simulink model "model_5"  (R2017b)
settings: Solver=ode3  StartTime=0.0  StopTime=4  FixedStep=2e-6  MaxStep=2e-05  RelTol=1e-3
undefined symbols (not defined in the file or in its folder): c1, c2_dot, c3_dot, c4_dot, J_10_dot, J_1_dot, J_2_dot, J_37_dot, J_810_dot, M_51new, M_52new, Mdnew, Mf10_mass5, Mf1_mass5, Mf2_mass5, Mf37_mass5, Mf810_mass5
libraries: fl_lib x29, nesl_utility x11, simulink x5
settings Model: Creator=Elena  LastModifiedBy=Elena
settings SolverCC: ZeroCrossAlgorithm=Adaptive
settings DebuggingCC: IgnoredZcDiagnostic=none
settings CodeAppCC: StateflowObjectComments=on

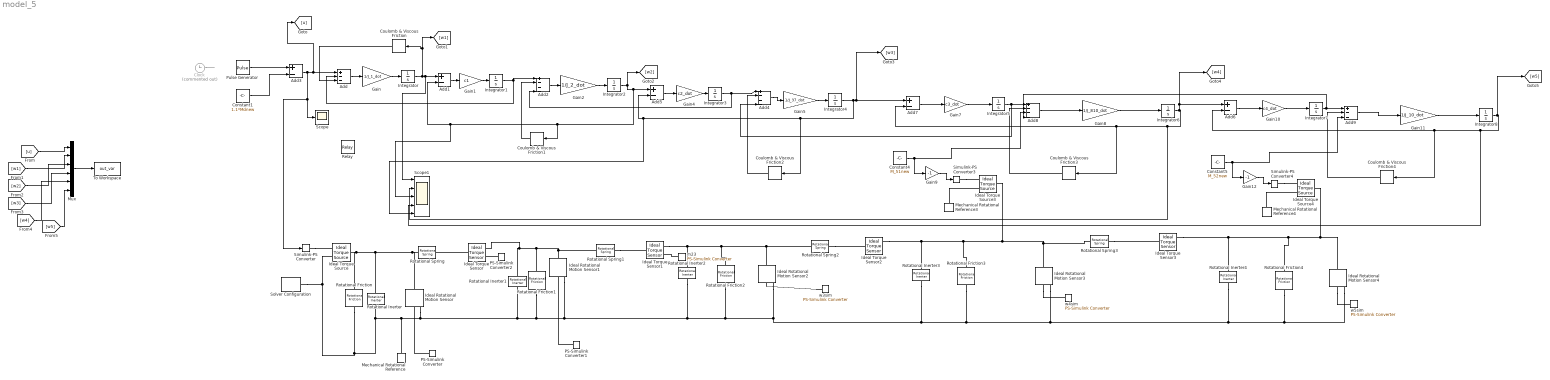
== system model_5 ==
  Add : Sum  Inputs=+--
  Add{1,3,5..7} (5 alike) : Sum  Inputs=+-
  Add2 : Sum  Inputs=+---
  Add4 : Sum  Inputs=+---
  Add8 : Sum  Inputs=+---
  Add9 : Sum  Inputs=+--
  Clock : Clock  Commented=on
  Constant1 : Constant  Value=1.1*Mdnew
  Constant4 : Constant  Value=M_51new
  Constant5 : Constant  Value=M_52new
  Coulomb & Viscous Friction : simulink/Discontinuities/Coulomb & Viscous Friction  offset=[Mf1_mass5]  gain=0
      settings: SourceProductName=Simulink
  Coulomb & Viscous Friction1 : simulink/Discontinuities/Coulomb & Viscous Friction  offset=[Mf2_mass5]  gain=0
      settings: SourceProductName=Simulink
  Coulomb & Viscous Friction2 : simulink/Discontinuities/Coulomb & Viscous Friction  offset=[Mf37_mass5]  gain=0
      settings: SourceProductName=Simulink
  Coulomb & Viscous Friction3 : simulink/Discontinuities/Coulomb & Viscous Friction  offset=[Mf810_mass5]  gain=0
      settings: SourceProductName=Simulink
  Coulomb & Viscous Friction4 : simulink/Discontinuities/Coulomb & Viscous Friction  offset=[Mf10_mass5]  gain=0
      settings: SourceProductName=Simulink
  Gain : Gain  Gain=1/J_1_dot
  Gain1 : Gain  Gain=c1
  Gain10 : Gain  Gain=c4_dot
  Gain11 : Gain  Gain=1/J_10_dot
  Gain12 : Gain  Gain=-1
  Gain2 : Gain  Gain=1/J_2_dot
  Gain4 : Gain  Gain=c2_dot
  Gain5 : Gain  Gain=1/J_37_dot
  Gain7 : Gain  Gain=c3_dot
  Gain8 : Gain  Gain=1/J_810_dot
  Gain9 : Gain  Gain=-1
  Ideal Rotational Motion Sensor{,1..4} (5 alike) : fl_lib/Mechanical/Mechanical Sensors/Ideal Rotational Motion Sensor  offset=0 rad
      settings: SourceProductBaseCode=PW,SS,VE
  Ideal Torque Sensor{,1..3} (4 alike) : fl_lib/Mechanical/Mechanical Sensors/Ideal Torque Sensor
      settings: SourceProductBaseCode=PW,SS,VE
  Ideal Torque Source : fl_lib/Mechanical/Mechanical Sources/Ideal Torque Source
      settings: SourceProductBaseCode=PW,SS,VE
  Ideal Torque Source3 : fl_lib/Mechanical/Mechanical Sources/Ideal Torque Source
      settings: SourceProductBaseCode=PW,SS,VE
  Ideal Torque Source4 : fl_lib/Mechanical/Mechanical Sources/Ideal Torque Source
      settings: SourceProductBaseCode=PW,SS,VE
  Integrator{,1..8} (9 alike) : Integrator
  Mechanical Rotational Reference : fl_lib/Mechanical/Rotational Elements/Mechanical Rotational Reference
      settings: SourceProductBaseCode=PW,SS,VE
  Mechanical Rotational Reference3 : fl_lib/Mechanical/Rotational Elements/Mechanical Rotational Reference
      settings: SourceProductBaseCode=PW,SS,VE
  Mechanical Rotational Reference4 : fl_lib/Mechanical/Rotational Elements/Mechanical Rotational Reference
      settings: SourceProductBaseCode=PW,SS,VE
  Mux : Mux  Inputs=6
  PS-Simulink Converter : nesl_utility/PS-Simulink Converter  PhysicalDomain=network_engine_domain  SubClassName=ps_output  LeftPortType=input  RightPortType=output  PseudoPeriodic=off  Frequencies=[]  Unit=rad/s  AffineConversion=off
      settings: SourceProductBaseCode=SS,PW,VE
  PS-Simulink Converter1 : nesl_utility/PS-Simulink Converter  PhysicalDomain=network_engine_domain  SubClassName=ps_output  LeftPortType=input  RightPortType=output  PseudoPeriodic=off  Frequencies=[]  Unit=rad/s  AffineConversion=off
      settings: SourceProductBaseCode=SS,PW,VE
  PS-Simulink Converter2 : nesl_utility/PS-Simulink Converter  PhysicalDomain=network_engine_domain  SubClassName=ps_output  LeftPortType=input  RightPortType=output  PseudoPeriodic=off  Frequencies=[]  Unit=N*m  AffineConversion=off
      settings: SourceProductBaseCode=SS,PW,VE
  Pulse Generator : DiscretePulseGenerator  PulseType=Time based  Amplitude=2.2*Mdnew  Period=1  PulseWidth=50
  Relay : Relay
  Rotational Friction : fl_lib/Mechanical/Rotational Elements/Rotational Friction  brkwy_trq=Mf1_mass5 N*m  brkwy_vel=1e-06 rad/s  Col_trq=Mf1_mass5 N*m  visc_coef=0 N*m/(rad/s)  w_specify=off  w_priority=None  w=0 rad/s  w_nominal_specify=off  w_nominal_unit=rad/s  w_nominal_value=1  t_specify=off  t_priority=None  t=0 N*m  t_nominal_specify=off  t_nominal_unit=N*m  t_nominal_value=1
      settings: SourceProductBaseCode=PW,SS,VE
  Rotational Friction1 : fl_lib/Mechanical/Rotational Elements/Rotational Friction  brkwy_trq=Mf2_mass5 N*m  brkwy_vel=1e-06 rad/s  Col_trq=Mf2_mass5 N*m  visc_coef=0 N*m/(rad/s)  w_specify=off  w_priority=None  w=0 rad/s  w_nominal_specify=off  w_nominal_unit=rad/s  w_nominal_value=1  t_specify=off  t_priority=None  t=0 N*m  t_nominal_specify=off  t_nominal_unit=N*m  t_nominal_value=1
      settings: SourceProductBaseCode=PW,SS,VE
  Rotational Friction2 : fl_lib/Mechanical/Rotational Elements/Rotational Friction  brkwy_trq=Mf37_mass5 N*m  brkwy_vel=1e-06 rad/s  Col_trq=Mf37_mass5 N*m  visc_coef=0 N*m/(rad/s)  w_specify=off  w_priority=None  w=0 rad/s  w_nominal_specify=off  w_nominal_unit=rad/s  w_nominal_value=1  t_specify=off  t_priority=None  t=0 N*m  t_nominal_specify=off  t_nominal_unit=N*m  t_nominal_value=1
      settings: SourceProductBaseCode=PW,SS,VE
  Rotational Friction3 : fl_lib/Mechanical/Rotational Elements/Rotational Friction  brkwy_trq=Mf810_mass5 N*m  brkwy_vel=1e-06 rad/s  Col_trq=Mf810_mass5 N*m  visc_coef=0 N*m/(rad/s)  w_specify=off  w_priority=None  w=0 rad/s  w_nominal_specify=off  w_nominal_unit=rad/s  w_nominal_value=1  t_specify=off  t_priority=None  t=0 N*m  t_nominal_specify=off  t_nominal_unit=N*m  t_nominal_value=1
      settings: SourceProductBaseCode=PW,SS,VE
  Rotational Friction4 : fl_lib/Mechanical/Rotational Elements/Rotational Friction  brkwy_trq=Mf10_mass5 N*m  brkwy_vel=1e-06 rad/s  Col_trq=Mf10_mass5 N*m  visc_coef=0 N*m/(rad/s)  w_specify=off  w_priority=None  w=0 rad/s  w_nominal_specify=off  w_nominal_unit=rad/s  w_nominal_value=1  t_specify=off  t_priority=None  t=0 N*m  t_nominal_specify=off  t_nominal_unit=N*m  t_nominal_value=1
      settings: SourceProductBaseCode=PW,SS,VE
  Rotational Inerter : fl_lib/Mechanical/Rotational Elements/Rotational Inerter  B=J_1_dot kg*m^2  w_specify=off  w_priority=High  w=0 rad/s  w_nominal_specify=off  w_nominal_unit=rad/s  w_nominal_value=1  t_specify=off  t_priority=None  t=0 N*m  t_nominal_specify=off  t_nominal_unit=N*m  t_nominal_value=1
      settings: SourceProductBaseCode=PW,SS,VE
  Rotational Inerter1 : fl_lib/Mechanical/Rotational Elements/Rotational Inerter  B=J_2_dot kg*m^2  w_specify=off  w_priority=High  w=0 rad/s  w_nominal_specify=off  w_nominal_unit=rad/s  w_nominal_value=1  t_specify=off  t_priority=None  t=0 N*m  t_nominal_specify=off  t_nominal_unit=N*m  t_nominal_value=1
      settings: SourceProductBaseCode=PW,SS,VE
  Rotational Inerter2 : fl_lib/Mechanical/Rotational Elements/Rotational Inerter  B=J_37_dot kg*m^2  w_specify=off  w_priority=High  w=0 rad/s  w_nominal_specify=off  w_nominal_unit=rad/s  w_nominal_value=1  t_specify=off  t_priority=None  t=0 N*m  t_nominal_specify=off  t_nominal_unit=N*m  t_nominal_value=1
      settings: SourceProductBaseCode=PW,SS,VE
  Rotational Inerter3 : fl_lib/Mechanical/Rotational Elements/Rotational Inerter  B=J_810_dot kg*m^2  w_specify=off  w_priority=High  w=0 rad/s  w_nominal_specify=off  w_nominal_unit=rad/s  w_nominal_value=1  t_specify=off  t_priority=None  t=0 N*m  t_nominal_specify=off  t_nominal_unit=N*m  t_nominal_value=1
      settings: SourceProductBaseCode=PW,SS,VE
  Rotational Inerter4 : fl_lib/Mechanical/Rotational Elements/Rotational Inerter  B=J_10_dot kg*m^2  w_specify=off  w_priority=High  w=0 rad/s  w_nominal_specify=off  w_nominal_unit=rad/s  w_nominal_value=1  t_specify=off  t_priority=None  t=0 N*m  t_nominal_specify=off  t_nominal_unit=N*m  t_nominal_value=1
      settings: SourceProductBaseCode=PW,SS,VE
  Rotational Spring : fl_lib/Mechanical/Rotational Elements/Rotational Spring  spr_rate=c1 N*m/rad  w_specify=off  w_priority=None  w=0 rad/s  w_nominal_specify=off  w_nominal_unit=rad/s  w_nominal_value=1  t_specify=off  t_priority=None  t=0 N*m  t_nominal_specify=off  t_nominal_unit=N*m  t_nominal_value=1  phi_specify=off  phi_priority=High  phi=0 rad  phi_nominal_specify=off  phi_nominal_unit=rad  phi_nominal_value=1
      settings: SourceProductBaseCode=PW,SS,VE
  Rotational Spring1 : fl_lib/Mechanical/Rotational Elements/Rotational Spring  spr_rate=c2_dot N*m/rad  w_specify=off  w_priority=None  w=0 rad/s  w_nominal_specify=off  w_nominal_unit=rad/s  w_nominal_value=1  t_specify=off  t_priority=None  t=0 N*m  t_nominal_specify=off  t_nominal_unit=N*m  t_nominal_value=1  phi_specify=off  phi_priority=High  phi=0 rad  phi_nominal_specify=off  phi_nominal_unit=rad  phi_nominal_value=1
      settings: SourceProductBaseCode=PW,SS,VE
  Rotational Spring2 : fl_lib/Mechanical/Rotational Elements/Rotational Spring  spr_rate=c3_dot N*m/rad  w_specify=off  w_priority=None  w=0 rad/s  w_nominal_specify=off  w_nominal_unit=rad/s  w_nominal_value=1  t_specify=off  t_priority=None  t=0 N*m  t_nominal_specify=off  t_nominal_unit=N*m  t_nominal_value=1  phi_specify=off  phi_priority=High  phi=0 rad  phi_nominal_specify=off  phi_nominal_unit=rad  phi_nominal_value=1
      settings: SourceProductBaseCode=PW,SS,VE
  Rotational Spring3 : fl_lib/Mechanical/Rotational Elements/Rotational Spring  spr_rate=c4_dot N*m/rad  w_specify=off  w_priority=None  w=0 rad/s  w_nominal_specify=off  w_nominal_unit=rad/s  w_nominal_value=1  t_specify=off  t_priority=None  t=0 N*m  t_nominal_specify=off  t_nominal_unit=N*m  t_nominal_value=1  phi_specify=off  phi_priority=High  phi=0 rad  phi_nominal_specify=off  phi_nominal_unit=rad  phi_nominal_value=1
      settings: SourceProductBaseCode=PW,SS,VE
  Scope : Scope
  Scope1 : Scope  NumInputPorts=5
  Simulink-PS Converter : nesl_utility/Simulink-PS Converter  PhysicalDomain=network_engine_domain  SubClassName=ps_input  LeftPortType=input  RightPortType=output  PseudoPeriodic=off  Frequencies=[]  NoiseDistribution=none  NoiseParameters=[]  Unit=1  AffineConversion=off  FilteringAndDerivatives=provide  SimscapeFilterOrder=1  InputFilterTimeConstant=2e-5  UdotUserProvided=0
      settings: SourceProductBaseCode=SS,PW,VE
  Simulink-PS Converter3 : nesl_utility/Simulink-PS Converter  PhysicalDomain=network_engine_domain  SubClassName=ps_input  LeftPortType=input  RightPortType=output  PseudoPeriodic=off  Frequencies=[]  NoiseDistribution=none  NoiseParameters=[]  Unit=1  AffineConversion=off  FilteringAndDerivatives=provide  SimscapeFilterOrder=1  InputFilterTimeConstant=0.001  UdotUserProvided=0
      settings: SourceProductBaseCode=SS,PW,VE
  Simulink-PS Converter4 : nesl_utility/Simulink-PS Converter  PhysicalDomain=network_engine_domain  SubClassName=ps_input  LeftPortType=input  RightPortType=output  PseudoPeriodic=off  Frequencies=[]  NoiseDistribution=none  NoiseParameters=[]  Unit=1  AffineConversion=off  FilteringAndDerivatives=provide  SimscapeFilterOrder=1  InputFilterTimeConstant=0.001  UdotUserProvided=0
      settings: SourceProductBaseCode=SS,PW,VE
  Solver Configuration : nesl_utility/Solver Configuration  PhysicalDomain=network_engine_domain  SubClassName=solver  LeftPortType=input  RightPortType=generic  Accelerate=off  Tones=[]  Harmonics=[]  SimulateNoise=off  Profile=off  UseLocalSampling=off  EnableSwitchedLinearOptims=on  FrequencyDomain=off  UseCCode=off  RelTol=0.001  AbsTol=1e-06  MinStep=1e-09  ToWorkspace=off  RevertToSquareIcSolve=off  NumHomotopyIterations=100  PhasorMode=off  PhasorModeNumHarmonics=1  DoDC=off  ResidualTolerance=1e-09  UseLocalSolver=on  LocalSolverChoice=NE_TRAPEZOIDAL_ADVANCER  LocalSolverSampleTime=1e-5  DoFixedCost=on  MaxNonlinIter=3  MaxModeIter=2  LinearAlgebra=Sparse  DelaysMemoryBudget=1024  AutomaticFiltering=on  FilteringTimeConstant=0.001
      settings: SourceProductBaseCode=SS,PW,VE
  To Workspace : ToWorkspace  VariableName=out_var  SaveFormat=Structure With Time  SampleTime=0.001
  m23 : nesl_utility/PS-Simulink Converter  PhysicalDomain=network_engine_domain  SubClassName=ps_output  LeftPortType=input  RightPortType=output  PseudoPeriodic=off  Frequencies=[]  Unit=N*m  AffineConversion=off
      settings: SourceProductBaseCode=SS,PW,VE
  w3sim : nesl_utility/PS-Simulink Converter  PhysicalDomain=network_engine_domain  SubClassName=ps_output  LeftPortType=input  RightPortType=output  PseudoPeriodic=off  Frequencies=[]  Unit=rad/s  AffineConversion=off
      settings: SourceProductBaseCode=SS,PW,VE
  w4sim : nesl_utility/PS-Simulink Converter  PhysicalDomain=network_engine_domain  SubClassName=ps_output  LeftPortType=input  RightPortType=output  PseudoPeriodic=off  Frequencies=[]  Unit=rad/s  AffineConversion=off
      settings: SourceProductBaseCode=SS,PW,VE
  w5sim : nesl_utility/PS-Simulink Converter  PhysicalDomain=network_engine_domain  SubClassName=ps_output  LeftPortType=input  RightPortType=output  PseudoPeriodic=off  Frequencies=[]  Unit=rad/s  AffineConversion=off
      settings: SourceProductBaseCode=SS,PW,VE
  wires:
  Gain/1 -> Integrator/1
  Gain1/1 -> Integrator1/1
  Gain2/1 -> Integrator2/1
  Add/1 -> Gain/1
  Pulse Generator/1 -> Add3/1
  Constant1/1 -> Add3/2
  Add3/1 -> Simulink-PS Converter/1, Scope/1, [u], Add/1
  Add1/1 -> Gain1/1
  Integrator1/1 -> Add/2, Add2/1
  Add2/1 -> Gain2/1
  Integrator2/1 -> Add5/1, Add1/2, Scope1/3, Coulomb & Viscous Friction1/1, [w2]
  Coulomb & Viscous Friction1/1 -> Add2/2
  Mux/1 -> To Workspace/1
  Integrator/1 -> Coulomb & Viscous Friction/1, [w1], Scope1/1, Add1/1
  [u] -> Mux/1
  [w1] -> Mux/2
  [w2] -> Mux/3
  Clock/1 -> ?
  Coulomb & Viscous Friction/1 -> Add/3
  Gain4/1 -> Integrator3/1
  Add5/1 -> Gain4/1
  Integrator3/1 -> Add2/4, Add4/1
  Add4/1 -> Gain5/1
  Gain5/1 -> Integrator4/1
  Integrator4/1 -> Add7/1, [w3], Coulomb & Viscous Friction2/1, Scope1/5, Add5/2
  Coulomb & Viscous Friction2/1 -> Add4/2
  [w3] -> Mux/4
  Add7/1 -> Gain7/1
  Gain7/1 -> Integrator5/1
  Integrator5/1 -> Add4/4, Add8/1
  Add8/1 -> Gain8/1
  Gain8/1 -> Integrator6/1
  Integrator6/1 -> Add6/1, [w4], Scope1/2, Coulomb & Viscous Friction3/1, Add7/2
  Gain9/1 -> Simulink-PS Converter3/1
  Coulomb & Viscous Friction3/1 -> Add8/2
  Constant4/1 -> Add8/3, Gain9/1
  [w4] -> Mux/5
  Integrator8/1 -> [w5], Scope1/4, Coulomb & Viscous Friction4/1, Add6/2
  Gain10/1 -> Integrator7/1
  Coulomb & Viscous Friction4/1 -> Add9/2
  Add6/1 -> Gain10/1
  Constant5/1 -> Add9/3, Gain12/1
  Add9/1 -> Gain11/1
  Integrator7/1 -> Add8/4, Add9/1
  Gain11/1 -> Integrator8/1
  Gain12/1 -> Simulink-PS Converter4/1
  [w5] -> Mux/6
  connections:
  Simulink-PS Converter/RConn1 -- Ideal Torque Source/RConn1
  Ideal Torque Source/LConn1 -- Rotational Friction/LConn1 -- Ideal Rotational Motion Sensor/LConn1 -- Rotational Spring/LConn1 -- Rotational Inerter/LConn1
  Mechanical Rotational Reference/LConn1 -- Ideal Rotational Motion Sensor/RConn1 -- Ideal Rotational Motion Sensor1/RConn1 -- Rotational Inerter2/RConn1 -- Rotational Friction4/RConn1 -- Ideal Rotational Motion Sensor4/RConn1 -- Rotational Inerter4/RConn1 -- Ideal Rotational Motion Sensor3/RConn1 -- Rotational Friction3/RConn1 -- Rotational Inerter3/RConn1 -- Ideal Rotational Motion Sensor2/RConn1 -- Rotational Friction2/RConn1 -- Rotational Friction1/RConn1 -- Rotational Inerter1/RConn1 -- Rotational Friction/RConn1 -- Solver Configuration/RConn1 -- Ideal Torque Source/RConn2 -- Rotational Inerter/RConn1
  Ideal Torque Sensor/LConn1 -- Rotational Spring/RConn1
  Ideal Torque Sensor/RConn1 -- Rotational Spring1/LConn1 -- Ideal Rotational Motion Sensor1/LConn1 -- Rotational Friction1/LConn1 -- Rotational Inerter1/LConn1
  PS-Simulink Converter/LConn1 -- Ideal Rotational Motion Sensor/RConn2
  PS-Simulink Converter1/LConn1 -- Ideal Rotational Motion Sensor1/RConn2
  PS-Simulink Converter2/LConn1 -- Ideal Torque Sensor/RConn2
  Rotational Spring1/RConn1 -- Ideal Torque Sensor1/LConn1
  Ideal Torque Sensor1/RConn1 -- Rotational Friction2/LConn1 -- Rotational Spring2/LConn1 -- Ideal Rotational Motion Sensor2/LConn1 -- Rotational Inerter2/LConn1
  w3sim/LConn1 -- Ideal Rotational Motion Sensor2/RConn2
  m23/LConn1 -- Ideal Torque Sensor1/RConn2
  Rotational Spring2/RConn1 -- Ideal Torque Sensor2/LConn1
  Ideal Torque Sensor2/RConn1 -- Ideal Torque Source3/LConn1 -- Rotational Spring3/LConn1 -- Ideal Rotational Motion Sensor3/LConn1 -- Rotational Friction3/LConn1 -- Rotational Inerter3/LConn1
  Simulink-PS Converter3/RConn1 -- Ideal Torque Source3/RConn1
  Ideal Torque Source3/RConn2 -- Mechanical Rotational Reference3/LConn1
  Ideal Torque Source4/RConn2 -- Mechanical Rotational Reference4/LConn1
  Simulink-PS Converter4/RConn1 -- Ideal Torque Source4/RConn1
  Rotational Spring3/RConn1 -- Ideal Torque Sensor3/LConn1
  Ideal Torque Sensor3/RConn1 -- Ideal Torque Source4/LConn1 -- Ideal Rotational Motion Sensor4/LConn1 -- Rotational Friction4/LConn1 -- Rotational Inerter4/LConn1
  Ideal Rotational Motion Sensor3/RConn2 -- w4sim/LConn1
  Ideal Rotational Motion Sensor4/RConn2 -- w5sim/LConn1
